simulink model "FM_Bistatic_Radar_V2"  (R2025a)
settings: Solver=VariableStepAuto  StartTime=0.0  StopTime=10.0  RelTol=1e-3
libraries: commchan3 x2, phaseddetectlib x1, dspadpt3 x1
settings Model: Creator=leifefrancisco  LastModifiedBy=leifefrancisco

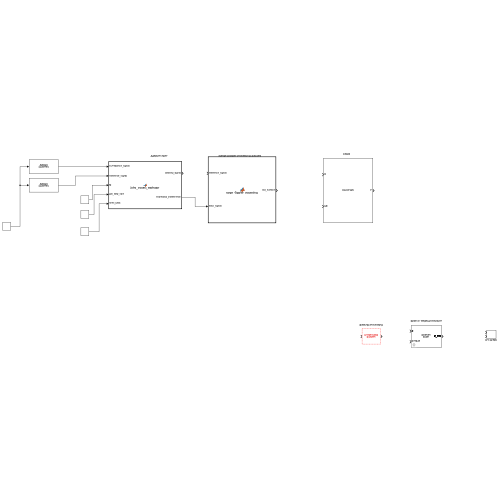
[thumbnail: Simulink's stored preview of the top-level diagram]
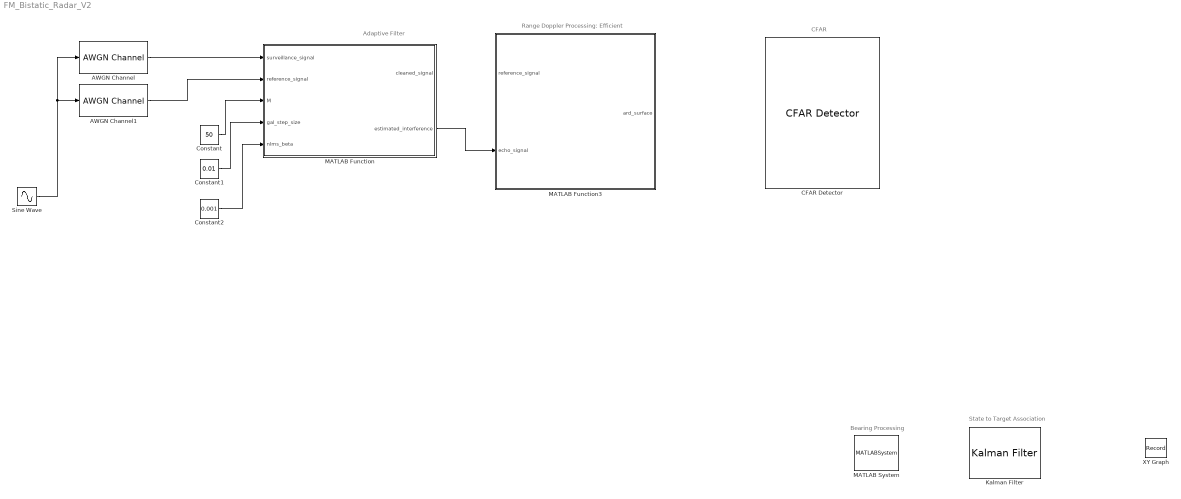
== system FM_Bistatic_Radar_V2 ==
  note: State to Target Association
  note: Bearing Processing
  note: CFAR
  note: Range Doppler Processing: Efficient
  note: Adaptive Filter
  AWGN Channel : commchan3/AWGN Channel  LegacyMode=off  NoiseMethod="Signal to noise ratio  (SNR)"  noiseMode="Signal to noise ratio  (SNR)"  EbNo=10  EsNo=10  SNR=-80  BitsPerSymbol=1  SignalPower=1  SpecifySymbolPeriod=off  SamplesPerSymbol=1  SymbolPeriod=1  VarianceSource=Parameter  Variance=1  RandomStream=Global stream  Seed=67  SimulateUsing=Code generation
  AWGN Channel1 : commchan3/AWGN Channel  LegacyMode=off  NoiseMethod="Signal to noise ratio  (SNR)"  noiseMode="Signal to noise ratio  (SNR)"  EbNo=10  EsNo=10  SNR=40  BitsPerSymbol=1  SignalPower=1  SpecifySymbolPeriod=off  SamplesPerSymbol=1  SymbolPeriod=1  VarianceSource=Parameter  Variance=1  RandomStream=Global stream  Seed=67  SimulateUsing=Code generation
  CFAR Detector : phaseddetectlib/CFAR Detector  Method=CA  Rank=1  NumGuardCells=2  NumTrainingCells=2  ThresholdFactor=Auto  ProbabilityFalseAlarm=0.1  CustomThresholdFactor=1  OutputFormat=CUT result  ThresholdOutputPort=off  NoisePowerOutputPort=off  NumDetectionsSource=Auto  NumDetections=1  SimulateUsing=Interpreted execution
  Constant : Constant  Value=50
  Constant1 : Constant  Value=0.01
  Constant2 : Constant  Value=0.001
  Kalman Filter : dspadpt3/Kalman Filter  num_targets=10  sourceEnable=Specify via input port <Enable>  isReset=on  X=zeros([6, 1])  P=10*eye(6)  A=[1 0 1 0 0 0;0 1 0 1 0 0; 0 0 1 0 0 0; 0 0 0 1 0 0; 0 0 0 0 1 0; 0 0 0 0 0 1]  sourceMeasure=Specify via dialog  H=[1 0 0 0 0 0; 0 1 0 0 0 0; 0 0 0 0 1 0; 0 0 0 0 0 1]  Q=0.05*eye(6)  R=eye(4)  isOutputEstMeasure=on  isOutputEstState=off  isOutputEstError=off  isOutputPrdMeasure=off  isOutputPrdState=off  isOutputPrdError=off
  MATLAB Function : MATLAB Function  TreatAsAtomicUnit=on
  MATLAB Function3 : MATLAB Function  TreatAsAtomicUnit=on
  MATLAB System : MATLABSystem
  Sine Wave : Sin  SampleTime=0
  XY Graph : Record  NumPorts=2.0  FileSettingsInternal="{\"entries\":[{\"content\":{\"excelSettings\":{\"content\":{},\"type\":\"Streamout.ExcelSettings\"},\"parquetSettings\":{\"content\":{},\"type\":\"Streamout.ParquetSettings\"}},\"type\":\"Streamout.FileSettingStorage\",\"uuid\":\"\"}],\"packageUris\":[\"http:\\/\\/schema.mathworks.com\\/mf0\\/streamout_blocks\\/R2020a\"],\"version\":\"1.0\"}"  FrameSettings=[0, 0]  Layout=[1 1]  SignalsInternal="{\"entries\":[{\"content\":{\"signals\":[{\"content\":{\"blockPath\":[],\"dimensions\":[1],\"domain\":\"\",\"lineColor\":\"#a2142f\",\"plots\":[ 1 ],\"port\":1,\"signalID\":1,\"signalName\":\"XY Graph:1\"},\"type\":\"RecordBlkView.Signal\",\"uuid\":\"\"},{\"content\":{\"blockPath\":[],\"dimensions\":[1],\"domain\":\"\",\"lineColor\":\"#139fff\",\"plots\":[ 1 ],\"port\":2,\"signalID\":2,\"signalName\":\"XY Graph:2\"},\"type\":\"RecordBlkView.Signal\",\"uuid\":\"\"}]},\"type\":\"RecordBlkView.InputSignals\",\"uuid\":\"\"}],\"packageUris\":[\"http:\\/\\/schema.mathworks.com\\/mf0\\/streamout_blocks\\/R2020a\"],\"version\":\"1.0\"}"  VisualizationBindings="{\"xyplotplugin\":{\"info\":[{\"series\":[{\"bindingParametersList\":[{\"parameter\":\"X-Axis\",\"signalID\":1,\"signalName\":\"XY Graph:1\"},{\"parameter\":\"Y-Axis\",\"signalID\":2,\"signalName\":\"XY Graph:2\"}],\"seriesID\":0}],\"subplotID\":1}]}}"  CompatibilityTag=XY
  wires:
  AWGN Channel/1 -> MATLAB Function/1(surveillance_signal)
  Constant/1 -> MATLAB Function/3(M)
  Constant1/1 -> MATLAB Function/4(gal_step_size)
  Constant2/1 -> MATLAB Function/5(nlms_beta)
  MATLAB Function/2(estimated_interference) -> MATLAB Function3/2(echo_signal)
  AWGN Channel1/1 -> MATLAB Function/2(reference_signal)
  Sine Wave/1 -> AWGN Channel/1, AWGN Channel1/1

== matlab function FM_Bistatic_Radar_V2/MATLAB Function ==
  data: surveillance_signal input; cleaned_signal output; reference_signal input; M input; gal_step_size input; nlms_beta input; estimated_interference output
function [cleaned_signal, estimated_interference] = joint_process_estimator(surveillance_signal, reference_signal, M, gal_step_size, nlms_beta)
% joint_process_estimator: Implements an adaptive noise canceller.
%
% Inputs:
%   surveillance_signal : The main input signal (e.g., noisy_bb_signal). This is x(n) in the paper's Fig. 5.
%   reference_signal    : The reference signal correlated with the interference. This is w2(n) in Fig. 5.
%   M                   : The order of the lattice filter (e.g., 50).
%   gal_step_size       : The learning rate for the GAL reflection coefficients (kappa).
%   nlms_beta           : The learning rate for the NLMS Tapped Delay Line weights (h).
%
% Outputs:
%   cleaned_signal      : The output signal after interference has been removed. This is e(n) in Fig. 5.
%   estimated_interference: The estimated interference signal produced by the TDL. This is w1_hat(n) in Fig. 5.

  % --- 1. Initialization (Happens ONCE, before the main loop) ---
  % State variables for the filter that will be updated over time.
  kappas = zeros(M, 1);      % A vector to hold all M reflection coefficients.
  h_vector = zeros(M + 1, 1); % A vector for the M+1 Tapped Delay Line weights (for b0 to bM).
  b_delayed = zeros(M + 1, 1); % The "notepad" for b_0(i-1) through b_M(i-1).
  delta = 1e-6; % Small constant for NLMS denominator to prevent division by zero.

  num_samples = length(surveillance_signal);
  % Create arrays to store the final results.
  cleaned_signal = zeros(size(surveillance_signal));
  estimated_interference = zeros(size(surveillance_signal));

  % --- 2. Main Time Loop (Processes the entire signal sample by sample) ---
  for i = 1:num_samples

      % --- Setup for the current time step 'i' ---
      ref_sample = reference_signal(i); % The input to the GAL is the reference signal.
      f_current = ref_sample;           % Initialize the temporary forward error with the reference sample, f_0(i).
      b_current_n = zeros(M + 1, 1);    % A *new blank notepad* for today's backward errors.
      b_current_n(1) = ref_sample;      % Store b_0(i).

      % --- 3. Inner Stage Loop (Processes one sample through all M GAL stages) ---
      for k = 1:M
          % Get the inputs for the current stage 'k'.
          f_input = f_current;                      % This is f_{k-1}(i).
          b_delayed_input = b_delayed(k);           % This is b_{k-1}(i-1) from our "notepad".
          kappa_k = kappas(k);                      % The current reflection coefficient for this stage.

          % Calculate new forward and backward errors for stage 'k'.
          f_new = f_input + conj(kappa_k) * b_delayed_input; % This is f_k(i).
          b_new = kappa_k * f_input + b_delayed_input;      % This is b_k(i).

          % Update the reflection coefficient for this stage for the NEXT time step.
          gradient = 2 * f_new * conj(b_delayed_input);
          kappas(k) = kappa_k - gal_step_size * gradient;

          % Prepare for the next stage in this inner loop by passing the forward error along.
          f_current = f_new;
          % Write the new backward error to today's notepad.
          b_current_n(k + 1) = b_new;
      end

      % --- 4. Tapped Delay Line (TDL) Logic ---
      % The inner GAL loop is now done. `b_current_n` holds all M+1 backward errors for time 'i'.
      % These are the inputs to the Tapped Delay Line.

      % A) Calculate the TDL output using the CURRENT weights (`h_vector`).
      %    This is the estimated interference for time 'i'.
      estimated_interference_i = h_vector' * b_current_n;

      % B) Calculate the final system error using the SURVEILLANCE signal sample.
      %    This is also the "cleaned" output signal for this time step.
      surveillance_sample = surveillance_signal(i);
      final_error_i = surveillance_sample - estimated_interference_i;

      % C) Update the TDL weights for the NEXT time step using the NLMS rule.
      input_power = sum(abs(b_current_n).^2);
      h_vector = h_vector + (nlms_beta / (delta + input_power)) * final_error_i * b_current_n;

      % --- 5. Store Final Outputs and Update State for Next Time Step ---
      cleaned_signal(i) = final_error_i;
      estimated_interference(i) = estimated_interference_i;

      % Update the GAL's "notepad" of delayed backward errors for the next time step.
      b_delayed = b_current_n;

  end % End of main time loop

end % End of function

== matlab function FM_Bistatic_Radar_V2/MATLAB Function3 ==
  data: reference_signal input; ard_surface output; echo_signal input
function ard_surface = range_doppler_processing(reference_signal, echo_signal)
  %first we find the product of the conjugated time delayed reference signal and the echo signal
  %a find the conjugate of the time delayed reference signal
  % i = length(reference_signal); %this is how we tell the for loop to stop MISTAKE
  % declare all the parameters
  %{
## ******------Parameters-----*********
## echo signal = e_n
## delayed signal = d_m_n
## decimation factor = R
## number of bins = n_b
## then you put that into a vector and build your surface
## Author: leife francisco  <leifefrancisco@Mac.attlocal.net>
## Created: 2025-06-25
%}
  e_n = echo_signal;
  d_n = reference_signal;
  %now find the number of range bins
  %find the range resolution
  range_resolution = (3e8)/2.4e6;
  num_range_bins = 150000/range_resolution;

  %now find the decimation factor
  %choosing the decimation face R <= sampling_frequency/(2*maximum_doppler_frequency)
  %the maximum_doppler_frequency is equal to the 2*velocity/wavlength*cos(theta).
  %Then based on this find R from the formula above just use a power of two.
  %maximum_velocity = 200; %900 km/hr or 200m/s which is like a commercial jet
  %wavelength = 3e8/108e6; % lambda = 3e8 (m/s)/(frequency) (1/s)
  %sampling_frequency = 2.4e6; %the sampling freq is 2.4 Ms/s
  %maximum_doppler_frequency = (2*maximum_velocity)/wavelength; % should be about 500
  %decimation_factor = floor(((log2((sampling_frequency/(2*maximum_doppler_frequency)));
  r=2^11;
  %r = 2^decimation_factor
  integration_time = 1; %we use an integration time of 1 second
  total_number_of_samples = sampling_frequency * integration_time;
  %now find the number of fast fourier transform points (I don't think points is the right word)
  n_f = total_number_of_samples/r;
  %actually now we declare the ARD surface
  ard_surface = zeros(n_f, num_range_bins);
  %now start our for loop. The for loop loops the entire length of the range bins
  for i=1:num_range_bins
  %okay we're inside the for loop
  %now find the produce of the delayed reference signal and the echo signal
    delayed_d_n = [zeros(1,i), d_n(1: end-i)];
    d_m_n = conj(delayed_d_n);
    s_n = d_m_n.*e_n; %product of the conjugated time delayed reference signal and echo signal
  %now decimate by using the CIC function
  %first we integrate using cumulative sum
    integrated_signal = cumsum(s_n);
    decimate_end = length(integrated_signal);
  %now we're going to decimate the integrated function
    s_d_n = integrated_signal(1:r:decimate_end);
    differentiated_signal = diff(s_d_n);
  %now we put it through the low pass filter
  %first we have to design the filter
    new_sampling_frequency = round(sampling_frequency/r);
    w_n = 300/(new_sampling_frequency/2);
    b = fir1(4, w_n);
    filtered_cic_signal = filter(b, 1, differentiated_signal);
  % now we do the fast fourier transform
    s_fft = fft(filtered_cic_signal);
  % now put this range doppler bin inside the ard_surface
    ard_surface(:, i) = abs(s_fft);
  % loop back
   end

endfunction
